simulink model "RapiroWalk"  (R2014a)
settings: Solver=ode3  SolverMode=SingleTasking  StartTime=0.0  StopTime=inf  RelTol=1e-3
libraries: arduinolib x5, simulink x4
settings Model: ExtModeTrigDuration=2  Creator=akaushik  LastModifiedBy=yanlianz
settings OptimizationCC: OptimizeModelRefInitCode=on  LifeSpan=1
settings DebuggingCC: UnderspecifiedInitializationDetection=Classic  SolverPrmCheckMsg=none
settings HardwareCC: ProdBitPerInt=16  ProdBitPerPointer=8  ProdIntDivRoundTo=Zero  ProdEndianess=LittleEndian  ProdWordSize=8  ProdHWDeviceType=Atmel->AVR
settings RTWCC: SystemTargetFile=realtime.tlc  GenerateMakefile=off  TemplateMakefile=realtime.tmf  Description=Run on Target Hardware  RTWVerbose=off  ProcessScript=realtime_make_rtw_hook
settings STFCustomTargetCC: TargetLibSuffix=.a  GenerateSampleERTMain=on  ConcurrentExecutionCompliant=off  GeneratePreprocessorConditionals=Use local settings  ERTCustomFileBanners=on  SupportNonInlinedSFcns=off  SupportVariableSizeSignals=on  MATLABClassNameForMDSCustomization=Simulink.SoftwareTarget.ERTCustomization  GRTInterface=off  SystemTargetFile=realtime.tlc
settings ERTTargetCC: CombineOutputUpdateFcns=off  SupportContinuousTime=on  SupportVariableSizeSignals=on  ExtModeTransport=3  ExtModeMexFile=ext_serial_win32_comm  ExtModeMexArgs=0 1 9600  ERTSrcFileBannerTemplate=realtime_code_template.cgt  ERTHdrFileBannerTemplate=realtime_code_template.cgt  ERTDataSrcFileTemplate=realtime_code_template.cgt  ERTDataHdrFileTemplate=realtime_code_template.cgt  ERTCustomFileTemplate=realtime_file_process.tlc

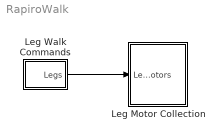
== system RapiroWalk ==
  Leg Motor Collection : Subsystem
  Leg Walk Commands : Subsystem
  wires:
  Leg Walk Commands/1(Legs) -> Leg Motor Collection/1(Leg_Motors)

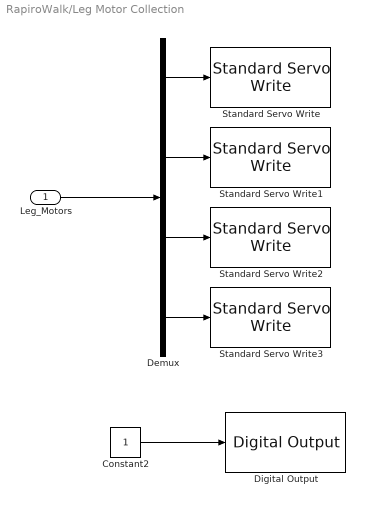
== system RapiroWalk/Leg Motor Collection ==
  Leg_Motors : Inport
  Constant2 : Constant
  Demux : Demux
  Digital Output : arduinolib/Digital Output  pinNumber=A3
  Standard Servo Write : arduinolib/Standard Servo Write  pinNumber=4
  Standard Servo Write1 : arduinolib/Standard Servo Write  pinNumber=2
  Standard Servo Write2 : arduinolib/Standard Servo Write  pinNumber=A1
  Standard Servo Write3 : arduinolib/Standard Servo Write  pinNumber=A2
  wires:
  Leg_Motors/1 -> Demux/1
  Demux/1 -> Standard Servo Write/1
  Demux/4 -> Standard Servo Write3/1
  Demux/2 -> Standard Servo Write1/1
  Demux/3 -> Standard Servo Write2/1
  Constant2/1 -> Digital Output/1

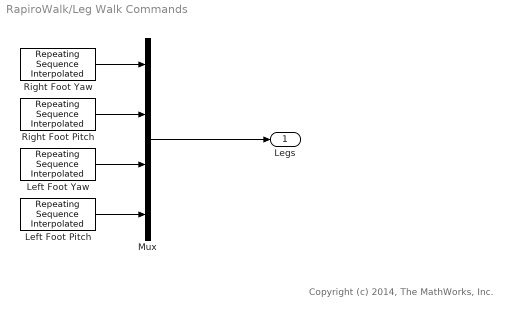
== system RapiroWalk/Leg Walk Commands ==
  note: Copyright (c) 2014, The MathWorks, Inc.
  Left Foot Pitch : simulink/Sources/Repeating Sequence Interpolated  OutValues=[120 90 80 70 90 110 120]  TimeValues=[0 1 2 3 4 5 6]*0.001  LookUpMeth=Interpolation-Use End Values  tsamp=0.000001  OutMin=[]  OutMax=[]  OutDataTypeStr=uint8  OutputDataTypeScalingMode=uint8  OutDataType=fixdt(0,8)  OutScaling=2^-10
  Left Foot Yaw : simulink/Sources/Repeating Sequence Interpolated  OutValues=[80 70 70 100 110 110 80]  TimeValues=[0 1 2 3 4 5 6]*0.001  LookUpMeth=Interpolation-Use End Values  tsamp=0.000001  OutMin=[]  OutMax=[]  OutDataTypeStr=uint8  OutputDataTypeScalingMode=uint8  OutDataType=fixdt(0,8)  OutScaling=2^-10
  Mux : Mux
  Right Foot Pitch : simulink/Sources/Repeating Sequence Interpolated  OutValues=[180 160 150 140 150 160 180]  TimeValues=[0 1 2 3 4 5 6]*0.001  LookUpMeth=Interpolation-Use End Values  tsamp=0.000001  OutMin=[]  OutMax=[]  OutDataTypeStr=uint8  OutputDataTypeScalingMode=uint8  OutDataType=fixdt(0,8)  OutScaling=2^-10
  Right Foot Yaw : simulink/Sources/Repeating Sequence Interpolated  OutValues=[80 70 70 100 110 110 80]  TimeValues=[0 1 2 3 4 5 6]*0.001  LookUpMeth=Interpolation-Use End Values  tsamp=0.000001  OutMin=[]  OutMax=[]  OutDataTypeStr=uint8  OutputDataTypeScalingMode=uint8  OutDataType=fixdt(0,8)  OutScaling=2^-10
  Legs : Outport
  wires:
  Left Foot Pitch/1 -> Mux/4
  Left Foot Yaw/1 -> Mux/3
  Right Foot Yaw/1 -> Mux/1
  Right Foot Pitch/1 -> Mux/2
  Mux/1 -> Legs/1
